simulink model "Pendulum_Native_2"  (R2021a)
settings: Solver=FixedStepDiscrete  StartTime=0.0  StopTime=inf  FixedStep=0.0050000000000000001  RelTol=1e-3
PostLoadFcn:
  | addpath(fileparts(get_param('Pendulum_Native_2','FileName')),fullfile(fileparts(get_param('Pendulum_Native_2','FileName')),'..','hardware'));
InitFcn:
  | addpath(fileparts(get_param('Pendulum_Native_2','FileName')),fullfile(fileparts(get_param('Pendulum_Native_2','FileName')),'..','hardware'));
settings Model: Creator=YW  LastModifiedBy=YW
settings DataIOCC: SaveOutput=off  SignalLogging=off  SaveTime=off
settings DebuggingCC: AlgebraicLoopMsg=error

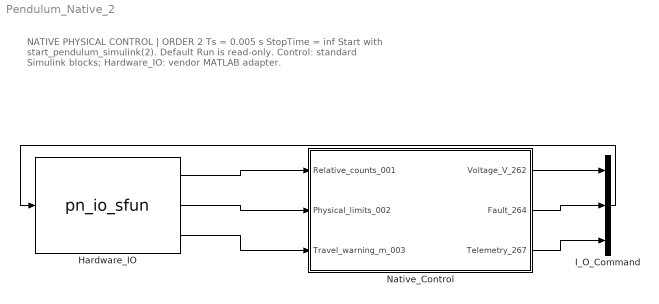
== system Pendulum_Native_2 ==
  note: NATIVE PHYSICAL CONTROL | ORDER 2
      | Ts = 0.005 s    StopTime = inf
      | Start with start_pendulum_simulink(2). Default Run is read-only.
      | Control: standard Simulink blocks; Hardware_IO: vendor MATLAB adapter.
  Hardware_IO : M-S-Function  FunctionName=pn_io_sfun  Parameters=2
  I_O_Command : Mux  Inputs=3
  Native_Control : Subsystem
  wires:
  Hardware_IO/1 -> Native_Control/1(Relative_counts_001)
  Hardware_IO/2 -> Native_Control/2(Physical_limits_002)
  Hardware_IO/3 -> Native_Control/3(Travel_warning_m_003)
  Native_Control/1(Voltage_V_262) -> I_O_Command/1
  Native_Control/2(Fault_264) -> I_O_Command/2
  Native_Control/3(Telemetry_267) -> I_O_Command/3
  I_O_Command/1 -> Hardware_IO/1

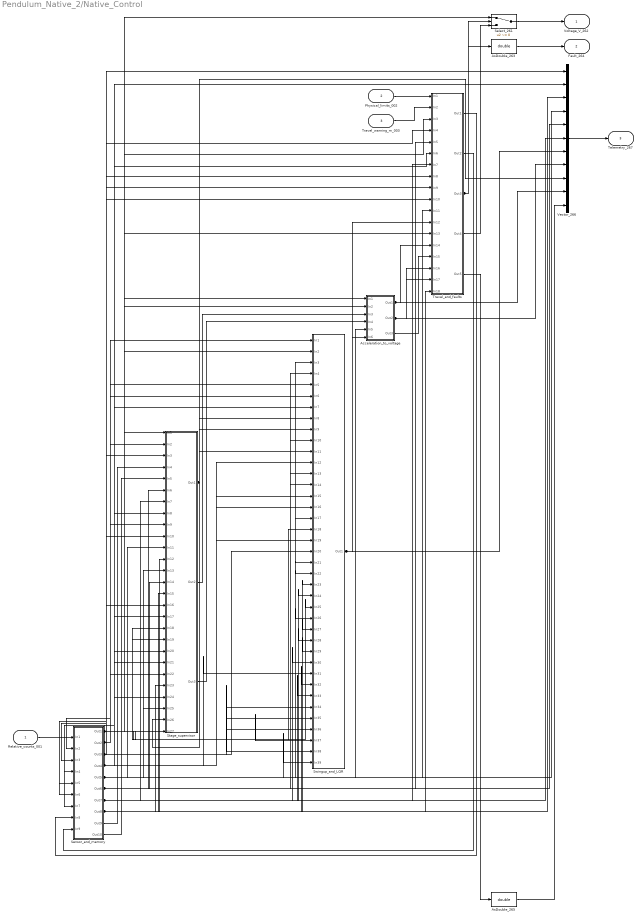
== system Pendulum_Native_2/Native_Control ==
  Relative_counts_001 : Inport  PortDimensions=3
  Physical_limits_002 : Inport  Port=2  PortDimensions=2
  Travel_warning_m_003 : Inport  Port=3  PortDimensions=1
  Acceleration_to_voltage : Subsystem
  AsDouble_263 : DataTypeConversion  OutDataTypeStr=double
  AsDouble_265 : DataTypeConversion  OutDataTypeStr=double
  Select_261 : Switch  Criteria=u2 ~= 0
  Sensor_and_memory : Subsystem
  Stage_supervisor : Subsystem
  Swingup_and_LQR : Subsystem
  Travel_and_faults : Subsystem
  Vector_266 : Mux  Inputs=11
  Voltage_V_262 : Outport
  Fault_264 : Outport  Port=2
  Telemetry_267 : Outport  Port=3
  wires:
  Travel_and_faults/1(Out1) -> Sensor_and_memory/8(In8)
  Stage_supervisor/3(Out3) -> Acceleration_to_voltage/4(In4)
  Travel_and_faults/5(Out5) -> AsDouble_265/1
  Travel_and_faults/2(Out2) -> Sensor_and_memory/9(In9)
  Travel_and_faults/4(Out4) -> Select_261/3
  Sensor_and_memory/4(Out4) -> Swingup_and_LQR/31(In31), Travel_and_faults/6(In6), Swingup_and_LQR/19(In19), Swingup_and_LQR/16(In16), Swingup_and_LQR/15(In15), Swingup_and_LQR/12(In12), Swingup_and_LQR/7(In7), Stage_supervisor/24(In24), Stage_supervisor/21(In21), Stage_supervisor/20(In20), Stage_supervisor/8(In8), Sensor_and_memory/7(In7), Vector_266/2, Stage_supervisor/17(In17), Sensor_and_memory/4(In4)
  Acceleration_to_voltage/3(Out3) -> Travel_and_faults/15(In15)
  Travel_warning_m_003/1 -> Travel_and_faults/2(In2)
  Physical_limits_002/1 -> Travel_and_faults/1(In1)
  Stage_supervisor/1(Out1) -> Swingup_and_LQR/8(In8), Vector_266/9, Swingup_and_LQR/9(In9), Stage_supervisor/26(In26), Swingup_and_LQR/11(In11)
  Stage_supervisor/2(Out2) -> Acceleration_to_voltage/3(In3)
  Sensor_and_memory/10(Out10) -> Stage_supervisor/5(In5)
  Sensor_and_memory/9(Out9) -> Stage_supervisor/4(In4)
  Relative_counts_001/1 -> Sensor_and_memory/1(In1)
  Sensor_and_memory/3(Out3) -> Swingup_and_LQR/38(In38), Travel_and_faults/10(In10), Swingup_and_LQR/35(In35), Swingup_and_LQR/34(In34), Travel_and_faults/8(In8), Swingup_and_LQR/20(In20), Stage_supervisor/3(In3), Stage_supervisor/10(In10), Travel_and_faults/4(In4), Swingup_and_LQR/36(In36), Travel_and_faults/9(In9), Sensor_and_memory/5(In5), Vector_266/1, Stage_supervisor/16(In16), Sensor_and_memory/6(In6), Sensor_and_memory/3(In3)
  Vector_266/1 -> Telemetry_267/1
  AsDouble_265/1 -> Vector_266/11
  AsDouble_263/1 -> Fault_264/1
  Select_261/1 -> Voltage_V_262/1
  Sensor_and_memory/6(Out6) -> Swingup_and_LQR/13(In13), Vector_266/5, Travel_and_faults/5(In5), Swingup_and_LQR/14(In14), Swingup_and_LQR/10(In10), Stage_supervisor/14(In14), Stage_supervisor/6(In6), Swingup_and_LQR/4(In4)
  Travel_and_faults/3(Out3) -> Select_261/2, AsDouble_263/1
  Acceleration_to_voltage/1(Out1) -> Vector_266/10, Travel_and_faults/14(In14)
  Acceleration_to_voltage/2(Out2) -> Vector_266/8, Travel_and_faults/17(In17), Travel_and_faults/16(In16)
  Swingup_and_LQR/1(Out1) -> Acceleration_to_voltage/6(In6), Travel_and_faults/12(In12), Vector_266/7
  Sensor_and_memory/5(Out5) -> Acceleration_to_voltage/5(In5), Travel_and_faults/11(In11), Swingup_and_LQR/39(In39), Swingup_and_LQR/22(In22), Swingup_and_LQR/26(In26), Vector_266/4, Swingup_and_LQR/17(In17), Swingup_and_LQR/21(In21), Stage_supervisor/13(In13), Stage_supervisor/25(In25), Stage_supervisor/11(In11), Swingup_and_LQR/3(In3)
  Sensor_and_memory/7(Out7) -> Vector_266/6, Travel_and_faults/7(In7), Swingup_and_LQR/33(In33), Swingup_and_LQR/30(In30), Swingup_and_LQR/28(In28), Swingup_and_LQR/24(In24), Stage_supervisor/7(In7)
  Sensor_and_memory/2(Out2) -> Stage_supervisor/9(In9), Swingup_and_LQR/5(In5), Sensor_and_memory/2(In2), Swingup_and_LQR/1(In1), Stage_supervisor/22(In22), Swingup_and_LQR/6(In6), Stage_supervisor/2(In2)
  Sensor_and_memory/8(Out8) -> Vector_266/3, Travel_and_faults/18(In18), Swingup_and_LQR/32(In32), Swingup_and_LQR/29(In29), Swingup_and_LQR/27(In27), Swingup_and_LQR/23(In23), Stage_supervisor/23(In23), Stage_supervisor/15(In15), Stage_supervisor/12(In12)
  Sensor_and_memory/1(Out1) -> Acceleration_to_voltage/1(In1), Travel_and_faults/13(In13), Swingup_and_LQR/25(In25), Stage_supervisor/18(In18), Acceleration_to_voltage/2(In2), Swingup_and_LQR/18(In18), Select_261/1, Swingup_and_LQR/37(In37), Swingup_and_LQR/2(In2), Stage_supervisor/27(In27), Stage_supervisor/1(In1), Stage_supervisor/19(In19), Travel_and_faults/3(In3)

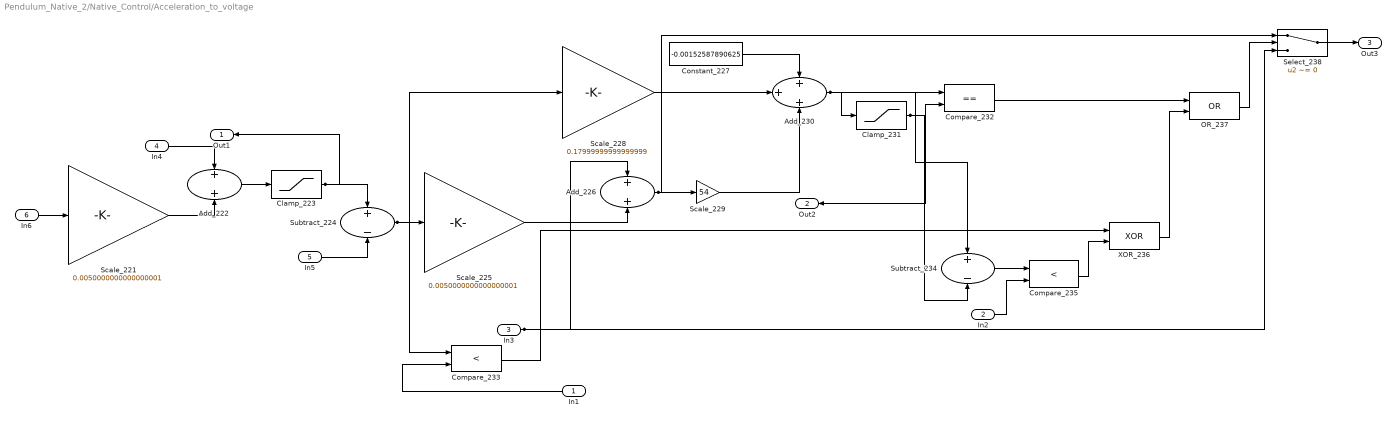
== system Pendulum_Native_2/Native_Control/Acceleration_to_voltage ==
  In1 : Inport
  In2 : Inport  Port=2
  In3 : Inport  Port=3
  In4 : Inport  Port=4
  In5 : Inport  Port=5
  In6 : Inport  Port=6
  Add_222 : Sum
  Add_226 : Sum
  Add_230 : Sum  Inputs=+++
  Clamp_223 : Saturate  UpperLimit=0.59999999999999998  LowerLimit=-0.59999999999999998
  Clamp_231 : Saturate  UpperLimit=1  LowerLimit=-1
  Compare_232 : RelationalOperator  Operator===  OutDataTypeStr=boolean  RndMeth=Simplest
  Compare_233 : RelationalOperator  Operator=<  OutDataTypeStr=boolean  RndMeth=Simplest
  Compare_235 : RelationalOperator  Operator=<  OutDataTypeStr=boolean  RndMeth=Simplest
  Constant_227 : Constant  Value=-0.00152587890625
  OR_237 : Logic  Operator=OR  AllPortsSameDT=off  OutDataTypeStr=boolean
  Scale_221 : Gain  Gain=0.0050000000000000001
  Scale_225 : Gain  Gain=0.0050000000000000001
  Scale_228 : Gain  Gain=0.17999999999999999
  Scale_229 : Gain  Gain=54
  Select_238 : Switch  Criteria=u2 ~= 0
  Subtract_224 : Sum  Inputs=+-
  Subtract_234 : Sum  Inputs=+-
  XOR_236 : Logic  Operator=XOR  AllPortsSameDT=off  OutDataTypeStr=boolean
  Out1 : Outport
  Out2 : Outport  Port=2
  Out3 : Outport  Port=3
  wires:
  Select_238/1 -> Out3/1
  Subtract_224/1 -> Scale_225/1, Scale_228/1, Compare_233/1
  In5/1 -> Subtract_224/2
  In1/1 -> Compare_233/2
  In6/1 -> Scale_221/1
  In2/1 -> Compare_235/2
  Scale_225/1 -> Add_226/2
  Clamp_223/1 -> Subtract_224/1, Out1/1
  Scale_221/1 -> Add_222/2
  Constant_227/1 -> Add_230/1
  OR_237/1 -> Select_238/2
  Add_222/1 -> Clamp_223/1
  Scale_229/1 -> Add_230/3
  In4/1 -> Add_222/1
  Compare_232/1 -> OR_237/1
  Scale_228/1 -> Add_230/2
  Subtract_234/1 -> Compare_235/1
  Compare_235/1 -> XOR_236/2
  Compare_233/1 -> XOR_236/1
  XOR_236/1 -> OR_237/2
  Clamp_231/1 -> Subtract_234/2, Out2/1, Compare_232/2
  In3/1 -> Add_226/1, Select_238/3
  Add_230/1 -> Clamp_231/1, Compare_232/1, Subtract_234/1
  Add_226/1 -> Scale_229/1, Select_238/1

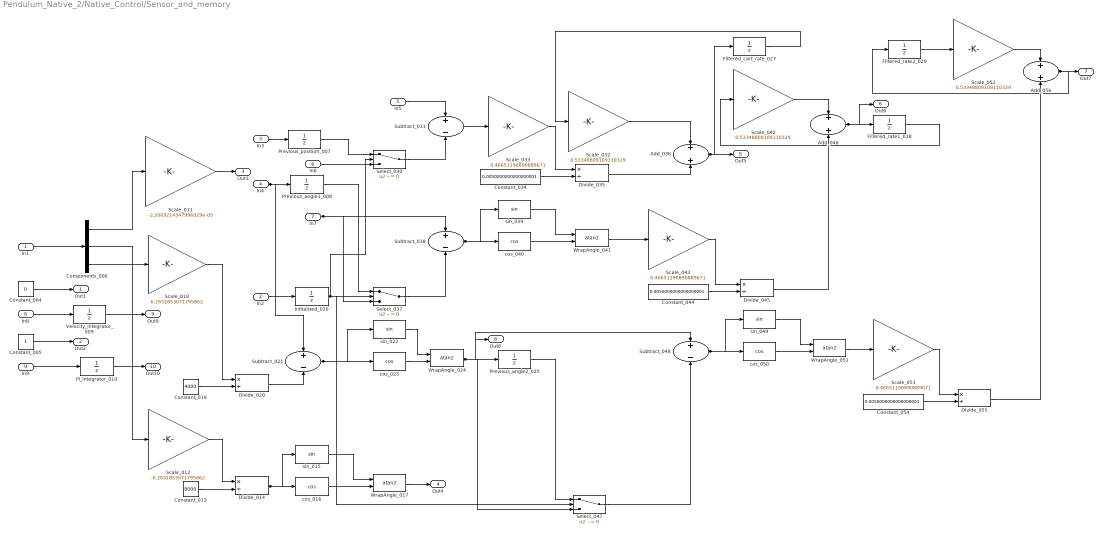
== system Pendulum_Native_2/Native_Control/Sensor_and_memory ==
  In1 : Inport
  In2 : Inport  Port=2
  In3 : Inport  Port=3
  In4 : Inport  Port=4
  In5 : Inport  Port=5
  In6 : Inport  Port=6
  In7 : Inport  Port=7
  In8 : Inport  Port=8
  In9 : Inport  Port=9
  Add_036 : Sum
  Add_046 : Sum
  Add_056 : Sum
  Components_006 : Demux  Outputs=3
  Constant_004 : Constant  Value=0
  Constant_005 : Constant
  Constant_013 : Constant  Value=8000
  Constant_019 : Constant  Value=4000
  Constant_034 : Constant  Value=0.0050000000000000001
  Constant_044 : Constant  Value=0.0050000000000000001
  Constant_054 : Constant  Value=0.0050000000000000001
  Divide_014 : Product  Inputs=*/
  Divide_020 : Product  Inputs=*/
  Divide_035 : Product  Inputs=*/
  Divide_045 : Product  Inputs=*/
  Divide_055 : Product  Inputs=*/
  Filtered_cart_rate_027 : UnitDelay  SampleTime=-1  HasFrameUpgradeWarning=on
  Filtered_rate1_028 : UnitDelay  SampleTime=-1  HasFrameUpgradeWarning=on
  Filtered_rate2_029 : UnitDelay  SampleTime=-1  HasFrameUpgradeWarning=on
  Initialized_026 : UnitDelay  SampleTime=-1  HasFrameUpgradeWarning=on
  PI_integrator_010 : UnitDelay  SampleTime=-1  HasFrameUpgradeWarning=on
  Previous_angle1_008 : UnitDelay  SampleTime=-1  HasFrameUpgradeWarning=on
  Previous_angle2_025 : UnitDelay  SampleTime=-1  HasFrameUpgradeWarning=on
  Previous_position_007 : UnitDelay  SampleTime=-1  HasFrameUpgradeWarning=on
  Scale_011 : Gain  Gain=-2.2069214347996029e-05
  Scale_012 : Gain  Gain=-6.2831853071795862
  Scale_018 : Gain  Gain=6.2831853071795862
  Scale_032 : Gain  Gain=0.53348809109110329
  Scale_033 : Gain  Gain=0.46651190890889671
  Scale_042 : Gain  Gain=0.53348809109110329
  Scale_043 : Gain  Gain=0.46651190890889671
  Scale_052 : Gain  Gain=0.53348809109110329
  Scale_053 : Gain  Gain=0.46651190890889671
  Select_030 : Switch  Criteria=u2 ~= 0
  Select_037 : Switch  Criteria=u2 ~= 0
  Select_047 : Switch  Criteria=u2 ~= 0
  Subtract_021 : Sum  Inputs=+-
  Subtract_031 : Sum  Inputs=+-
  Subtract_038 : Sum  Inputs=+-
  Subtract_048 : Sum  Inputs=+-
  Velocity_integrator_009 : UnitDelay  SampleTime=-1  HasFrameUpgradeWarning=on
  WrapAngle_017 : Trigonometry  Operator=atan2
  WrapAngle_024 : Trigonometry  Operator=atan2
  WrapAngle_041 : Trigonometry  Operator=atan2
  WrapAngle_051 : Trigonometry  Operator=atan2
  cos_016 : Trigonometry  Operator=cos
  cos_023 : Trigonometry  Operator=cos
  cos_040 : Trigonometry  Operator=cos
  cos_050 : Trigonometry  Operator=cos
  sin_015 : Trigonometry
  sin_022 : Trigonometry
  sin_039 : Trigonometry
  sin_049 : Trigonometry
  Out1 : Outport
  Out2 : Outport  Port=2
  Out3 : Outport  Port=3
  Out4 : Outport  Port=4
  Out5 : Outport  Port=5
  Out6 : Outport  Port=6
  Out7 : Outport  Port=7
  Out8 : Outport  Port=8
  Out9 : Outport  Port=9
  Out10 : Outport  Port=10
  wires:
  Velocity_integrator_009/1 -> Out9/1
  Scale_042/1 -> Add_046/1
  Scale_012/1 -> Divide_014/1
  In2/1 -> Initialized_026/1
  Subtract_031/1 -> Scale_033/1
  sin_022/1 -> WrapAngle_024/1
  WrapAngle_051/1 -> Scale_053/1
  cos_016/1 -> WrapAngle_017/2
  Select_037/1 -> Subtract_038/2
  PI_integrator_010/1 -> Out10/1
  In4/1 -> Subtract_021/1, Previous_angle1_008/1
  In8/1 -> Velocity_integrator_009/1
  WrapAngle_017/1 -> Out4/1
  Constant_004/1 -> Out1/1
  Filtered_rate2_029/1 -> Scale_052/1
  In5/1 -> Subtract_031/1
  Constant_013/1 -> Divide_014/2
  Divide_045/1 -> Add_046/2
  Components_006/1 -> Scale_011/1
  Divide_020/1 -> Subtract_021/2
  Components_006/2 -> Scale_012/1
  Constant_019/1 -> Divide_020/2
  Constant_005/1 -> Out2/1
  Filtered_rate1_028/1 -> Scale_042/1
  Divide_035/1 -> Add_036/2
  Previous_position_007/1 -> Select_030/1
  In9/1 -> PI_integrator_010/1
  cos_050/1 -> WrapAngle_051/2
  In3/1 -> Previous_position_007/1
  sin_039/1 -> WrapAngle_041/1
  Scale_018/1 -> Divide_020/1
  Scale_032/1 -> Add_036/1
  sin_049/1 -> WrapAngle_051/1
  Constant_044/1 -> Divide_045/2
  In6/1 -> Select_030/3
  Divide_014/1 -> sin_015/1, cos_016/1
  Divide_055/1 -> Add_056/2
  Select_047/1 -> Subtract_048/2
  Previous_angle2_025/1 -> Select_047/1
  cos_040/1 -> WrapAngle_041/2
  Add_036/1 -> Out5/1, Filtered_cart_rate_027/1
  Previous_angle1_008/1 -> Select_037/1
  cos_023/1 -> WrapAngle_024/2
  Filtered_cart_rate_027/1 -> Scale_032/1
  Constant_054/1 -> Divide_055/2
  WrapAngle_041/1 -> Scale_043/1
  Scale_011/1 -> Out3/1
  sin_015/1 -> WrapAngle_017/1
  WrapAngle_024/1 -> Select_047/3, Out8/1, Previous_angle2_025/1, Subtract_048/1
  Scale_053/1 -> Divide_055/1
  Subtract_048/1 -> sin_049/1, cos_050/1
  Scale_033/1 -> Divide_035/1
  Components_006/3 -> Scale_018/1
  Constant_034/1 -> Divide_035/2
  In7/1 -> Select_037/3, Subtract_038/1
  In1/1 -> Components_006/1
  Scale_043/1 -> Divide_045/1
  Scale_052/1 -> Add_056/1
  Add_056/1 -> Out7/1, Filtered_rate2_029/1
  Select_030/1 -> Subtract_031/2
  Add_046/1 -> Out6/1, Filtered_rate1_028/1
  Subtract_021/1 -> sin_022/1, cos_023/1
  Subtract_038/1 -> sin_039/1, cos_040/1
  Initialized_026/1 -> Select_037/2, Select_047/2, Select_030/2

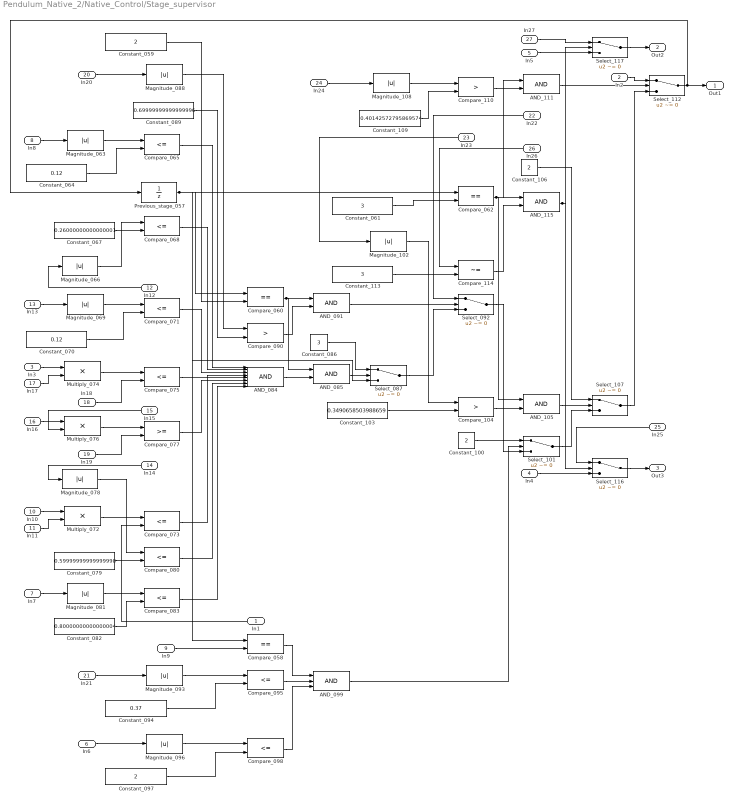
== system Pendulum_Native_2/Native_Control/Stage_supervisor ==
  In1 : Inport
  In2 : Inport  Port=2
  In3 : Inport  Port=3
  In4 : Inport  Port=4
  In5 : Inport  Port=5
  In6 : Inport  Port=6
  In7 : Inport  Port=7
  In8 : Inport  Port=8
  In9 : Inport  Port=9
  In10 : Inport  Port=10
  In11 : Inport  Port=11
  In12 : Inport  Port=12
  In13 : Inport  Port=13
  In14 : Inport  Port=14
  In15 : Inport  Port=15
  In16 : Inport  Port=16
  In17 : Inport  Port=17
  In18 : Inport  Port=18
  In19 : Inport  Port=19
  In20 : Inport  Port=20
  In21 : Inport  Port=21
  In22 : Inport  Port=22
  In23 : Inport  Port=23
  In24 : Inport  Port=24
  In25 : Inport  Port=25
  In26 : Inport  Port=26
  In27 : Inport  Port=27
  AND_084 : Logic  Inputs=8  AllPortsSameDT=off  OutDataTypeStr=boolean
  AND_085 : Logic  AllPortsSameDT=off  OutDataTypeStr=boolean
  AND_091 : Logic  AllPortsSameDT=off  OutDataTypeStr=boolean
  AND_099 : Logic  Inputs=3  AllPortsSameDT=off  OutDataTypeStr=boolean
  AND_105 : Logic  AllPortsSameDT=off  OutDataTypeStr=boolean
  AND_111 : Logic  AllPortsSameDT=off  OutDataTypeStr=boolean
  AND_115 : Logic  AllPortsSameDT=off  OutDataTypeStr=boolean
  Compare_058 : RelationalOperator  Operator===  OutDataTypeStr=boolean  RndMeth=Simplest
  Compare_060 : RelationalOperator  Operator===  OutDataTypeStr=boolean  RndMeth=Simplest
  Compare_062 : RelationalOperator  Operator===  OutDataTypeStr=boolean  RndMeth=Simplest
  Compare_065 : RelationalOperator  Operator=<=  OutDataTypeStr=boolean  RndMeth=Simplest
  Compare_068 : RelationalOperator  Operator=<=  OutDataTypeStr=boolean  RndMeth=Simplest
  Compare_071 : RelationalOperator  Operator=<=  OutDataTypeStr=boolean  RndMeth=Simplest
  Compare_073 : RelationalOperator  Operator=<=  OutDataTypeStr=boolean  RndMeth=Simplest
  Compare_075 : RelationalOperator  Operator=<=  OutDataTypeStr=boolean  RndMeth=Simplest
  Compare_077 : RelationalOperator  OutDataTypeStr=boolean  RndMeth=Simplest
  Compare_080 : RelationalOperator  Operator=<=  OutDataTypeStr=boolean  RndMeth=Simplest
  Compare_083 : RelationalOperator  Operator=<=  OutDataTypeStr=boolean  RndMeth=Simplest
  Compare_090 : RelationalOperator  Operator=>  OutDataTypeStr=boolean  RndMeth=Simplest
  Compare_095 : RelationalOperator  Operator=<=  OutDataTypeStr=boolean  RndMeth=Simplest
  Compare_098 : RelationalOperator  Operator=<=  OutDataTypeStr=boolean  RndMeth=Simplest
  Compare_104 : RelationalOperator  Operator=>  OutDataTypeStr=boolean  RndMeth=Simplest
  Compare_110 : RelationalOperator  Operator=>  OutDataTypeStr=boolean  RndMeth=Simplest
  Compare_114 : RelationalOperator  Operator=~=  OutDataTypeStr=boolean  RndMeth=Simplest
  Constant_059 : Constant  Value=2
  Constant_061 : Constant  Value=3
  Constant_064 : Constant  Value=0.12
  Constant_067 : Constant  Value=0.26000000000000001
  Constant_070 : Constant  Value=0.12
  Constant_079 : Constant  Value=0.59999999999999998
  Constant_082 : Constant  Value=0.80000000000000004
  Constant_086 : Constant  Value=3
  Constant_089 : Constant  Value=0.69999999999999996
  Constant_094 : Constant  Value=0.37
  Constant_097 : Constant  Value=2
  Constant_100 : Constant  Value=2
  Constant_103 : Constant  Value=0.3490658503988659
  Constant_106 : Constant  Value=2
  Constant_109 : Constant  Value=0.40142572795869574
  Constant_113 : Constant  Value=3
  Magnitude_063 : Abs
  Magnitude_066 : Abs
  Magnitude_069 : Abs
  Magnitude_078 : Abs
  Magnitude_081 : Abs
  Magnitude_088 : Abs
  Magnitude_093 : Abs
  Magnitude_096 : Abs
  Magnitude_102 : Abs
  Magnitude_108 : Abs
  Multiply_072 : Product
  Multiply_074 : Product
  Multiply_076 : Product
  Previous_stage_057 : UnitDelay  InitialCondition=1  SampleTime=-1  HasFrameUpgradeWarning=on
  Select_087 : Switch  Criteria=u2 ~= 0
  Select_092 : Switch  Criteria=u2 ~= 0
  Select_{101,107,112,116..117} (5 alike) : Switch  Criteria=u2 ~= 0
  Out1 : Outport
  Out2 : Outport  Port=2
  Out3 : Outport  Port=3
  wires:
  In27/1 -> Select_117/1
  In22/1 -> Select_092/1
  Magnitude_088/1 -> Compare_090/1
  In19/1 -> Compare_077/2
  In2/1 -> Select_112/1
  Constant_086/1 -> Select_087/1
  In11/1 -> Multiply_072/2
  In15/1 -> Multiply_076/2
  In4/1 -> Select_116/3
  Select_117/1 -> Out2/1
  AND_105/1 -> Select_107/2
  In10/1 -> Multiply_072/1
  In8/1 -> Magnitude_063/1
  Select_116/1 -> Out3/1
  In1/1 -> Compare_073/2
  In25/1 -> Select_116/1
  Compare_060/1 -> AND_085/1, AND_091/1
  Compare_075/1 -> AND_084/5
  In16/1 -> Multiply_076/1
  In17/1 -> Multiply_074/2
  Constant_079/1 -> Compare_080/2
  In14/1 -> Magnitude_078/1
  Compare_062/1 -> AND_105/1, AND_115/1, AND_111/1
  In3/1 -> Multiply_074/1
  In24/1 -> Magnitude_108/1
  Compare_058/1 -> AND_099/1
  In5/1 -> Select_117/3
  AND_084/1 -> AND_085/2
  In18/1 -> Compare_075/2
  Constant_082/1 -> Compare_083/2
  In12/1 -> Magnitude_066/1
  In21/1 -> Magnitude_093/1
  In13/1 -> Magnitude_069/1
  Compare_098/1 -> AND_099/3
  Multiply_076/1 -> Compare_077/1
  Magnitude_069/1 -> Compare_071/1
  Compare_073/1 -> AND_084/4
  Magnitude_081/1 -> Compare_083/1
  AND_111/1 -> Select_112/2
  Select_107/1 -> Select_112/3
  Compare_095/1 -> AND_099/2
  Compare_077/1 -> AND_084/6
  Multiply_074/1 -> Compare_075/1
  Compare_110/1 -> AND_111/2
  Compare_083/1 -> AND_084/8
  Compare_068/1 -> AND_084/2
  Magnitude_102/1 -> Compare_104/1
  Select_112/1 -> Out1/1, Previous_stage_057/1
  AND_085/1 -> Select_087/2
  Multiply_072/1 -> Compare_073/1
  Select_101/1 -> Select_107/3
  Constant_070/1 -> Compare_071/2
  In9/1 -> Compare_058/2
  Magnitude_078/1 -> Compare_080/1
  AND_091/1 -> Select_092/2
  Constant_113/1 -> Compare_114/2
  Magnitude_063/1 -> Compare_065/1
  Constant_059/1 -> Compare_060/2
  In26/1 -> Compare_114/1
  Magnitude_066/1 -> Compare_068/1
  Compare_090/1 -> AND_091/2
  Magnitude_093/1 -> Compare_095/1
  Magnitude_108/1 -> Compare_110/1
  Select_087/1 -> Select_092/3
  AND_099/1 -> Select_101/2
  Constant_106/1 -> Select_107/1
  Constant_109/1 -> Compare_110/2
  Constant_100/1 -> Select_101/1
  Constant_094/1 -> Compare_095/2
  Compare_104/1 -> AND_105/2
  Compare_065/1 -> AND_084/1
  Constant_097/1 -> Compare_098/2
  In23/1 -> Magnitude_102/1
  Constant_067/1 -> Compare_068/2
  In6/1 -> Magnitude_096/1
  Constant_103/1 -> Compare_104/2
  Constant_061/1 -> Compare_062/2
  Constant_064/1 -> Compare_065/2
  Magnitude_096/1 -> Compare_098/1
  Compare_071/1 -> AND_084/3
  Compare_114/1 -> AND_115/2
  Compare_080/1 -> AND_084/7
  Constant_089/1 -> Compare_090/2
  AND_115/1 -> Select_116/2, Select_117/2
  In7/1 -> Magnitude_081/1
  Select_092/1 -> Select_101/3
  In20/1 -> Magnitude_088/1
  Previous_stage_057/1 -> Compare_060/1, Compare_062/1, Select_087/3, Compare_058/1

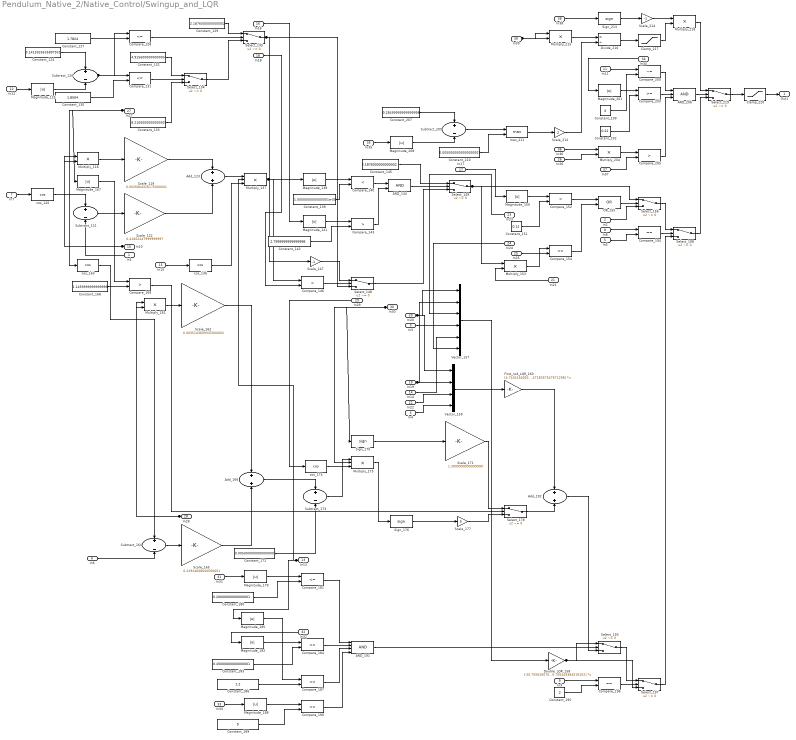
== system Pendulum_Native_2/Native_Control/Swingup_and_LQR ==
  In1 : Inport
  In2 : Inport  Port=2
  In3 : Inport  Port=3
  In4 : Inport  Port=4
  In5 : Inport  Port=5
  In6 : Inport  Port=6
  In7 : Inport  Port=7
  In8 : Inport  Port=8
  In9 : Inport  Port=9
  In10 : Inport  Port=10
  In11 : Inport  Port=11
  In12 : Inport  Port=12
  In13 : Inport  Port=13
  In14 : Inport  Port=14
  In15 : Inport  Port=15
  In16 : Inport  Port=16
  In17 : Inport  Port=17
  In18 : Inport  Port=18
  In19 : Inport  Port=19
  In20 : Inport  Port=20
  In21 : Inport  Port=21
  In22 : Inport  Port=22
  In23 : Inport  Port=23
  In24 : Inport  Port=24
  In25 : Inport  Port=25
  In26 : Inport  Port=26
  In27 : Inport  Port=27
  In28 : Inport  Port=28
  In29 : Inport  Port=29
  In30 : Inport  Port=30
  In31 : Inport  Port=31
  In32 : Inport  Port=32
  In33 : Inport  Port=33
  In34 : Inport  Port=34
  In35 : Inport  Port=35
  In36 : Inport  Port=36
  In37 : Inport  Port=37
  In38 : Inport  Port=38
  In39 : Inport  Port=39
  AND_144 : Logic  AllPortsSameDT=off  OutDataTypeStr=boolean
  AND_191 : Logic  Inputs=4  AllPortsSameDT=off  OutDataTypeStr=boolean
  AND_206 : Logic  Inputs=3  AllPortsSameDT=off  OutDataTypeStr=boolean
  Add_123 : Sum
  Add_166 : Sum
  Add_192 : Sum
  Clamp_217 : Saturate  UpperLimit=30  LowerLimit=2
  Clamp_220 : Saturate  UpperLimit=30  LowerLimit=-30
  Compare_{128,131,154,181,184,187,190} (7 alike) : RelationalOperator  Operator=<=  OutDataTypeStr=boolean  RndMeth=Simplest
  Compare_140 : RelationalOperator  Operator=<  OutDataTypeStr=boolean  RndMeth=Simplest
  Compare_{143,146,169,205} (4 alike) : RelationalOperator  Operator=>  OutDataTypeStr=boolean  RndMeth=Simplest
  Compare_152 : RelationalOperator  Operator=<  OutDataTypeStr=boolean  RndMeth=Simplest
  Compare_194 : RelationalOperator  Operator===  OutDataTypeStr=boolean  RndMeth=Simplest
  Compare_196 : RelationalOperator  Operator===  OutDataTypeStr=boolean  RndMeth=Simplest
  Compare_200 : RelationalOperator  Operator=~=  OutDataTypeStr=boolean  RndMeth=Simplest
  Compare_203 : RelationalOperator  OutDataTypeStr=boolean  RndMeth=Simplest
  Constant_124 : Constant  Value=3.1415926535897931
  Constant_127 : Constant  Value=1.7824
  Constant_129 : Constant  Value=2.1876000000000002
  Constant_130 : Constant  Value=1.8504
  Constant_132 : Constant  Value=4.9156000000000004
  Constant_133 : Constant  Value=8.2100000000000009
  Constant_139 : Constant  Value=1.0000000000000001e-09
  Constant_142 : Constant  Value=2.7999999999999998
  Constant_145 : Constant  Value=2.1876000000000002
  Constant_151 : Constant  Value=0.12
  Constant_168 : Constant  Value=1.1459999999999999
  Constant_172 : Constant  Value=0.0050000000000000001
  Constant_180 : Constant  Value=0.20000000000000001
  Constant_183 : Constant  Value=0.45000000000000001
  Constant_186 : Constant  Value=1.2
  Constant_189 : Constant  Value=9
  Constant_195 : Constant  Value=2
  Constant_199 : Constant  Value=3
  Constant_202 : Constant  Value=0.22
  Constant_207 : Constant  Value=0.28499999999999998
  Constant_210 : Constant  Value=0.0050000000000000001
  Divide_216 : Product  Inputs=*/
  Double_LQR_158 : Gain  Gain=[-20.755626070279462 -136.68455751706179 254.85837173801795 -24.440647335478328 -3.3044801353394511 40.750449384516202]  Multiplication=Matrix(K*u)
  First_rod_LQR_160 : Gain  Gain=[4.7434164902525744 -59.170534176527148 6.5584718328315059 -5.4718267547671298]  Multiplication=Matrix(K*u)
  Magnitude_{125,138,141,150,167,179,182,185,188,201,208} (11 alike) : Abs
  Multiply_{118,153,161,204,215,218} (6 alike) : Product
  Multiply_137 : Product  Inputs=3
  Multiply_175 : Product  Inputs=3
  OR_155 : Logic  Operator=OR  AllPortsSameDT=off  OutDataTypeStr=boolean
  Scale_119 : Gain  Gain=0.0025804316175000001
  Scale_122 : Gain  Gain=0.41602247999999997
  Scale_147 : Gain  Gain=-1
  Scale_162 : Gain  Gain=0.0035143609335000002
  Scale_165 : Gain  Gain=0.22924008000000001
  Scale_171 : Gain  Gain=1.3999999999999999
  Scale_177 : Gain  Gain=5
  Scale_212 : Gain  Gain=2
  Scale_214 : Gain  Gain=-1
  Select_{134..135,148..149,156,178,193,197..198,219} (10 alike) : Switch  Criteria=u2 ~= 0
  Sign_170 : Signum
  Sign_176 : Signum
  Sign_213 : Signum
  Subtract_{121,126,164,173,209} (5 alike) : Sum  Inputs=+-
  Vector_157 : Mux  Inputs=6
  Vector_159 : Mux
  cos_{120,136,163,174} (4 alike) : Trigonometry  Operator=cos
  max_211 : MinMax  Function=max  Inputs=2
  Out1 : Outport
  wires:
  In32/1 -> Magnitude_182/1
  In31/1 -> Magnitude_179/1
  Constant_151/1 -> Compare_152/2
  In33/1 -> Magnitude_188/1
  In35/1 -> Magnitude_208/1
  In24/1 -> Vector_157/6
  Magnitude_201/1 -> Compare_203/1
  Magnitude_150/1 -> Compare_152/1
  max_211/1 -> Scale_212/1
  In5/1 -> Compare_194/2
  Constant_202/1 -> Compare_203/2
  In8/1 -> Compare_194/1
  Compare_143/1 -> AND_144/2
  Constant_189/1 -> Compare_190/2
  In9/1 -> Compare_196/1
  In34/1 -> Magnitude_201/1
  In37/1 -> Compare_205/2
  In23/1 -> Vector_157/3
  In11/1 -> Compare_200/1
  Select_134/1 -> Select_135/3
  In22/1 -> Vector_159/3
  Compare_154/1 -> OR_155/2
  In3/1 -> Vector_157/4
  Magnitude_179/1 -> Compare_181/1
  In6/1 -> Subtract_164/2
  Constant_210/1 -> max_211/2
  Scale_122/1 -> Add_123/2
  In16/1 -> Magnitude_141/1
  Select_219/1 -> Clamp_220/1
  Constant_199/1 -> Compare_200/2
  In18/1 -> Compare_146/2
  In1/1 -> Subtract_121/2
  Compare_140/1 -> AND_144/1
  In15/1 -> cos_136/1
  Vector_159/1 -> First_rod_LQR_160/1
  In7/1 -> cos_120/1
  Subtract_209/1 -> max_211/1
  In2/1 -> Select_156/3
  In38/1 -> Sign_213/1
  In26/1 -> Multiply_204/2
  In36/1 -> Multiply_204/1
  In25/1 -> Compare_154/2
  In12/1 -> Magnitude_125/1
  In21/1 -> Multiply_153/2
  Magnitude_208/1 -> Subtract_209/2
  Compare_203/1 -> AND_206/2
  Compare_200/1 -> AND_206/1
  Magnitude_167/1 -> Compare_169/1
  Magnitude_182/1 -> Compare_184/1
  cos_120/1 -> Subtract_121/1
  In14/1 -> Vector_157/5
  Magnitude_141/1 -> Compare_143/1
  Compare_152/1 -> OR_155/1
  In17/1 -> Magnitude_150/1
  Constant_195/1 -> Compare_196/2
  Select_156/1 -> Select_198/1
  Constant_130/1 -> Compare_131/2
  Constant_172/1 -> Subtract_173/2
  Constant_139/1 -> Compare_140/2
  Constant_168/1 -> Compare_169/2
  AND_144/1 -> Select_149/2
  Magnitude_185/1 -> Compare_187/1
  In4/1 -> Vector_159/4
  cos_163/1 -> Subtract_164/1
  OR_155/1 -> Select_156/2
  Select_148/1 -> Select_149/3
  Compare_194/1 -> Select_198/2
  Constant_180/1 -> Compare_181/2
  Compare_181/1 -> AND_191/1
  Constant_145/1 -> Select_149/1
  Sign_176/1 -> Scale_177/1
  Compare_187/1 -> AND_191/3
  Add_192/1 -> Select_193/3
  Compare_190/1 -> AND_191/4
  Clamp_220/1 -> Out1/1
  Magnitude_138/1 -> Compare_140/1
  AND_191/1 -> Select_193/2
  Compare_196/1 -> Select_197/2
  Constant_142/1 -> Compare_143/2
  Constant_132/1 -> Select_134/1
  Compare_131/1 -> Select_134/2
  Add_123/1 -> Multiply_137/1
  Constant_127/1 -> Compare_128/2
  AND_206/1 -> Select_219/2
  cos_136/1 -> Multiply_137/3
  Compare_205/1 -> AND_206/3
  Multiply_215/1 -> Divide_216/1
  Clamp_217/1 -> Multiply_218/2
  cos_174/1 -> Multiply_175/3
  Multiply_204/1 -> Compare_205/1
  Subtract_173/1 -> Multiply_175/1
  Select_198/1 -> Select_219/3
  Multiply_218/1 -> Select_219/1
  Constant_183/1 -> Compare_184/2
  Constant_124/1 -> Subtract_126/1
  Scale_165/1 -> Add_166/2
  Scale_177/1 -> Select_178/3
  Sign_213/1 -> Scale_214/1
  Constant_133/1 -> Select_134/3
  Scale_212/1 -> Divide_216/2
  Compare_169/1 -> Select_178/2
  Scale_171/1 -> Select_178/1
  Constant_129/1 -> Select_135/1
  Multiply_161/1 -> Scale_162/1
  Select_178/1 -> Add_192/2
  Multiply_118/1 -> Scale_119/1
  Add_166/1 -> Subtract_173/1
  Compare_146/1 -> Select_148/2
  Constant_186/1 -> Compare_187/2
  Subtract_164/1 -> Scale_165/1
  In10/1 -> Multiply_118/1, Multiply_118/2
  Divide_216/1 -> Clamp_217/1
  Scale_119/1 -> Add_123/1
  Select_197/1 -> Select_198/3
  Scale_162/1 -> Add_166/1
  Constant_207/1 -> Subtract_209/1
  Scale_147/1 -> Select_148/1
  First_rod_LQR_160/1 -> Add_192/1
  Magnitude_188/1 -> Compare_190/1
  Scale_214/1 -> Multiply_218/1
  Magnitude_125/1 -> Subtract_126/2
  Sign_170/1 -> Scale_171/1
  Multiply_153/1 -> Compare_154/1
  Compare_184/1 -> AND_191/2
  Multiply_175/1 -> Sign_176/1
  Vector_157/1 -> Double_LQR_158/1
  Select_193/1 -> Select_197/1
  Compare_128/1 -> Select_135/2
  Subtract_121/1 -> Scale_122/1
  In29/1 -> cos_174/1
  In19/1 -> Vector_159/2, Vector_157/2
  Subtract_126/1 -> Compare_128/1, Compare_131/1
  In30/1 -> Sign_170/1, Multiply_175/2
  Multiply_137/1 -> Magnitude_138/1, Compare_146/1
  Select_149/1 -> Multiply_153/1, Select_156/1
  In13/1 -> Multiply_137/2, Magnitude_185/1
  In20/1 -> Vector_157/1, Vector_159/1
  Double_LQR_158/1 -> Select_193/1, Select_197/3
  In28/1 -> Multiply_161/2, Multiply_161/1
  In27/1 -> cos_163/1, Magnitude_167/1
  Select_135/1 -> Scale_147/1, Select_148/3
  In39/1 -> Multiply_215/1, Multiply_215/2

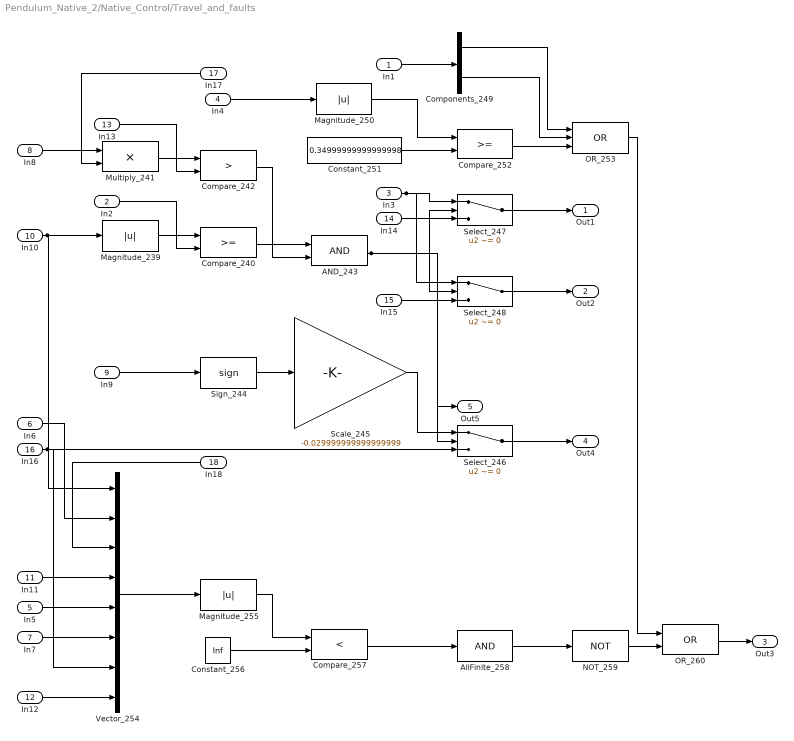
== system Pendulum_Native_2/Native_Control/Travel_and_faults ==
  In1 : Inport
  In2 : Inport  Port=2
  In3 : Inport  Port=3
  In4 : Inport  Port=4
  In5 : Inport  Port=5
  In6 : Inport  Port=6
  In7 : Inport  Port=7
  In8 : Inport  Port=8
  In9 : Inport  Port=9
  In10 : Inport  Port=10
  In11 : Inport  Port=11
  In12 : Inport  Port=12
  In13 : Inport  Port=13
  In14 : Inport  Port=14
  In15 : Inport  Port=15
  In16 : Inport  Port=16
  In17 : Inport  Port=17
  In18 : Inport  Port=18
  AND_243 : Logic  AllPortsSameDT=off  OutDataTypeStr=boolean
  AllFinite_258 : Logic  Inputs=1  AllPortsSameDT=off  OutDataTypeStr=boolean
  Compare_240 : RelationalOperator  OutDataTypeStr=boolean  RndMeth=Simplest
  Compare_242 : RelationalOperator  Operator=>  OutDataTypeStr=boolean  RndMeth=Simplest
  Compare_252 : RelationalOperator  OutDataTypeStr=boolean  RndMeth=Simplest
  Compare_257 : RelationalOperator  Operator=<  OutDataTypeStr=boolean  RndMeth=Simplest
  Components_249 : Demux  Outputs=2
  Constant_251 : Constant  Value=0.34999999999999998
  Constant_256 : Constant  Value=Inf
  Magnitude_239 : Abs
  Magnitude_250 : Abs
  Magnitude_255 : Abs
  Multiply_241 : Product
  NOT_259 : Logic  Operator=NOT  Inputs=1  AllPortsSameDT=off  OutDataTypeStr=boolean
  OR_253 : Logic  Operator=OR  Inputs=3  AllPortsSameDT=off  OutDataTypeStr=boolean
  OR_260 : Logic  Operator=OR  AllPortsSameDT=off  OutDataTypeStr=boolean
  Scale_245 : Gain  Gain=-0.029999999999999999
  Select_246 : Switch  Criteria=u2 ~= 0
  Select_247 : Switch  Criteria=u2 ~= 0
  Select_248 : Switch  Criteria=u2 ~= 0
  Sign_244 : Signum
  Vector_254 : Mux  Inputs=8
  Out1 : Outport
  Out2 : Outport  Port=2
  Out3 : Outport  Port=3
  Out4 : Outport  Port=4
  Out5 : Outport  Port=5
  wires:
  NOT_259/1 -> OR_260/2
  Compare_242/1 -> AND_243/2
  In2/1 -> Compare_240/2
  Vector_254/1 -> Magnitude_255/1
  Select_247/1 -> Out1/1
  In7/1 -> Vector_254/6
  In14/1 -> Select_247/3
  OR_260/1 -> Out3/1
  In9/1 -> Sign_244/1
  In1/1 -> Components_249/1
  Select_248/1 -> Out2/1
  In18/1 -> Vector_254/3
  In11/1 -> Vector_254/4
  Magnitude_239/1 -> Compare_240/1
  AllFinite_258/1 -> NOT_259/1
  OR_253/1 -> OR_260/1
  Components_249/2 -> OR_253/2
  In15/1 -> Select_248/3
  Components_249/1 -> OR_253/1
  Magnitude_255/1 -> Compare_257/1
  In10/1 -> Magnitude_239/1, Vector_254/1
  In5/1 -> Vector_254/5
  Select_246/1 -> Out4/1
  Magnitude_250/1 -> Compare_252/1
  Sign_244/1 -> Scale_245/1
  In13/1 -> Compare_242/2
  In17/1 -> Multiply_241/2
  In6/1 -> Vector_254/2
  In4/1 -> Magnitude_250/1
  Constant_256/1 -> Compare_257/2
  In8/1 -> Multiply_241/1
  Scale_245/1 -> Select_246/1
  Compare_257/1 -> AllFinite_258/1
  Compare_240/1 -> AND_243/1
  Constant_251/1 -> Compare_252/2
  In12/1 -> Vector_254/8
  Compare_252/1 -> OR_253/3
  Multiply_241/1 -> Compare_242/1
  In3/1 -> Select_248/1, Select_247/1
  AND_243/1 -> Select_247/2, Select_248/2, Select_246/2, Out5/1
  In16/1 -> Select_246/3, Vector_254/7
